simulink model "controllers"  (R2023a)
settings: Solver=VariableStepAuto  StartTime=0.0  StopTime=8e-3  RelTol=1e-3
libraries: simulink x1, spspowerguiLib x1
settings Model: Creator=pc180  LastModifiedBy=pc180

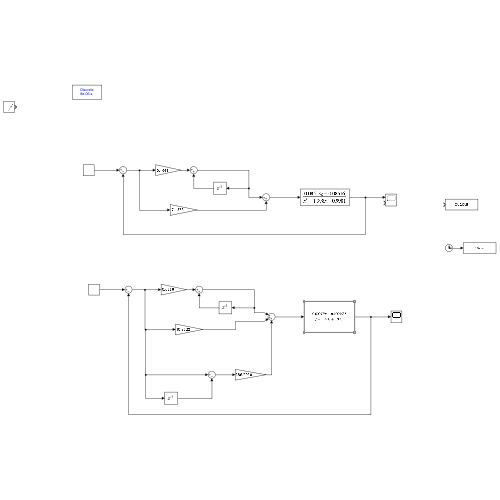
[thumbnail: Simulink's stored preview of the top-level diagram]
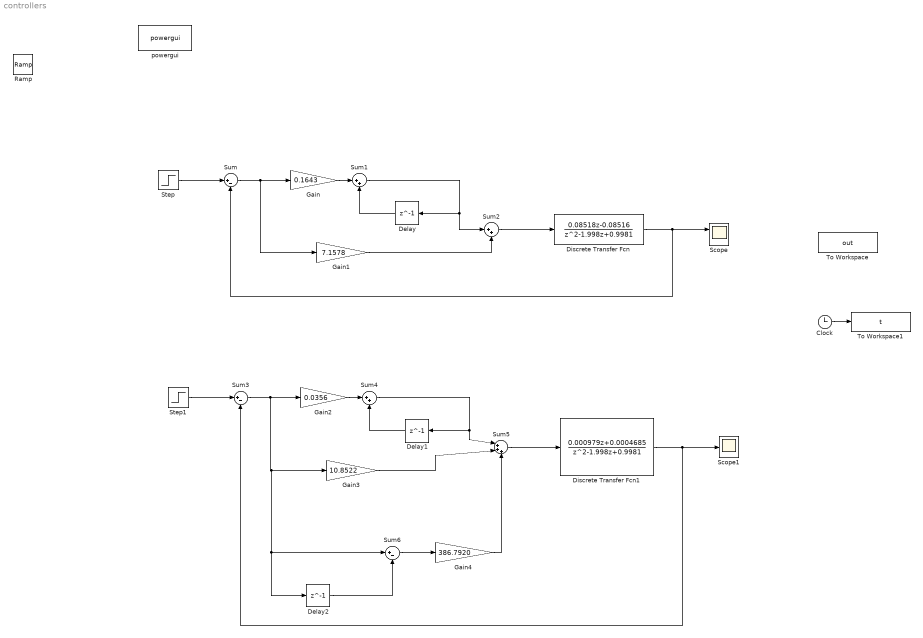
== system controllers ==
  Clock : Clock
  Delay : Delay  DelayLength=1  InitialCondition=0  SampleTime=8e-6
  Delay1 : Delay  DelayLength=1  InitialCondition=0  SampleTime=8e-6
  Delay2 : Delay  DelayLength=1  InitialCondition=0  SampleTime=8e-6
  Discrete Transfer Fcn : DiscreteTransferFcn  Numerator=[0.08518 -0.08516]  Denominator=[1 -1.998 0.9981]
  Discrete Transfer Fcn1 : DiscreteTransferFcn  Numerator=[0.000979 0.0004685]  Denominator=[1 -1.998 0.9981]  SampleTime=8e-6
  Gain : Gain  Gain=0.1643
  Gain1 : Gain  Gain=7.1578
  Gain2 : Gain  Gain=0.0356
  Gain3 : Gain  Gain=10.8522
  Gain4 : Gain  Gain=386.7920
  Ramp : simulink/Sources/Ramp  slope=0.5  start=0  InitialOutput=0
  Scope : Scope  NumInputPorts=2
  Scope1 : Scope
  Step : Step  Time=1e-3  SampleTime=8e-6
  Step1 : Step  Time=1e-3  SampleTime=8e-6
  Sum : Sum  Inputs=|+-
  Sum1 : Sum  Inputs=|++
  Sum2 : Sum  Inputs=|++
  Sum3 : Sum  Inputs=|+-
  Sum4 : Sum  Inputs=|++
  Sum5 : Sum  Inputs=|+++
  Sum6 : Sum  Inputs=|+-
  To Workspace : ToWorkspace  VariableName=out  SaveFormat=Timeseries  SampleTime=8e-6
  To Workspace1 : ToWorkspace  VariableName=t  SaveFormat=Timeseries  SampleTime=8e-6
  powergui : spspowerguiLib/powergui  Priority=1  SimulationMode=Discrete  SampleTime=8e-6  frequency=60  Iterations=50  frequencyindice=60  Pbase=100e6  ErrMax=1e-4  UnitsV=kV  UnitsW=MW  buscounter=0  FunctionMessages=off  echomessages=off  EnableUseOfTLC=off  CurrentSourceSwitches=off  DisableSnubberDevices=off  DisableRonSwitches=off  DisableVfSwitches=off  DisplayEquations=off  AutomaticDiscreteSolvers=off  SolverType=Tustin/Backward Euler (TBE)  Interpol=off  ExternalGateDelay=off  methode=off  Ts=100  x0status=blocks  SPID=on  SwTol=0  HookPort=off  NonlinearTolerance=1e-4  nMaxIteration=100  ContinueOnMaxIteration=off  RestoreLinks=warning  ResistiveCurrentMeasurement=off  Frange=[0:2:500]  Ylog=off  Xlog=on  ShowGrid=off  save=off  variable=ZData  structure=0  ZoomFFT=off  StartTime=0.0  cycles=1  DisplayStyle=1  fundamental=60  FreqAxis=off  MaxFrequency=1000  frequencyindicesteady=1  RmsSteady=1  display=off
  wires:
  Gain1/1 -> Sum2/2
  Sum1/1 -> Delay/1, Sum2/1
  Gain/1 -> Sum1/1
  Sum/1 -> Gain1/1, Gain/1
  Sum2/1 -> Discrete Transfer Fcn/1
  Delay/1 -> Sum1/2
  Discrete Transfer Fcn/1 -> Scope/1, Sum/2
  Step/1 -> Sum/1
  Step1/1 -> Sum3/1
  Gain2/1 -> Sum4/1
  Sum3/1 -> Delay2/1, Sum6/1, Gain3/1, Gain2/1
  Sum4/1 -> Delay1/1, Sum5/1
  Delay1/1 -> Sum4/2
  Sum5/1 -> Discrete Transfer Fcn1/1
  Discrete Transfer Fcn1/1 -> Scope1/1, Sum3/2
  Gain3/1 -> Sum5/2
  Delay2/1 -> Sum6/2
  Sum6/1 -> Gain4/1
  Gain4/1 -> Sum5/3
  Clock/1 -> To Workspace1/1
